simulink model "fullVehicleModel_17b"  (R2017b)
settings: Solver=VariableStepAuto  StartTime=0.0  StopTime=10.0  RelTol=1e-3
undefined symbols (not defined in the file): ambient_temp, bat, bat_r1, Batt, batt_initCharge, Batt_sensorLag_s, bvatt_AhRating, DiscIntNeverNeededParam, electronics_power, env, module_broad_area, module_small_area, module_top_area, mot, no_module, shifterPos, Ts, Ts_elec
libraries: Soft_ECUs x90, fl_lib x67, nesl_utility x29, Battery_lib x28, Gen_lib x13, simulink x10, aerolibconvert2 x7, SoftCAN_Interface x6, autolibshared x2, Additional_blocks_lib x1, elec_lib x1
(part 4 of 4)

== system fullVehicleModel_17b/Vehicle Model/Variant Subsystem/Subsystem/Battery Thermal/Module 5 ==
  Power Cycle : Inport
  Ideal Heat Flow Source : fl_lib/Thermal/Thermal Sources/Controlled Heat Flow Rate Source
      settings: SourceProductName=Simscape
  Ideal Temperature Sensor : fl_lib/Thermal/Thermal Sensors/Temperature Sensor
  Simulink-PS Converter1 : nesl_utility/Simulink-PS Converter  PhysicalDomain=network_engine_domain  SubClassName=ps_input  LeftPortType=input  RightPortType=output  PseudoPeriodic=off  Frequencies=[]  NoiseDistribution=none  NoiseParameters=[]  Unit=1  AffineConversion=off  FilteringAndDerivatives=zero  SimscapeFilterOrder=1  InputFilterTimeConstant=0.001  UdotUserProvided=1
  Thermal Mass : fl_lib/Thermal/Thermal Elements/Thermal Mass  mass=module_mass kg  sp_heat=specific_heat_module J/kg/K  T_specify=on  T_priority=High  T=ambient_temp K  T_nominal_specify=off  T_nominal_unit=K  T_nominal_value=1  Q_specify=off  Q_priority=High  Q=0 J/s  Q_nominal_specify=off  Q_nominal_unit=W  Q_nominal_value=1
  Thermal Reference1 : fl_lib/Thermal/Thermal Elements/Thermal Reference
  Thermal Reference2 : fl_lib/Thermal/Thermal Elements/Thermal Reference
  Temperature : PMIOPort  Port=1  Side=Right
  Air Convection : PMIOPort  Port=2  Side=Right
  Module to Module Convection : PMIOPort  Port=3  Side=Left
  Electronics to Module Convection : PMIOPort  Port=4  Side=Left
  wires:
  Power Cycle/1 -> Simulink-PS Converter1/1
  connections:
  Ideal Heat Flow Source/RConn1 -- Simulink-PS Converter1/RConn1
  Thermal Reference2/LConn1 -- Ideal Heat Flow Source/RConn2
  Temperature/RConn1 -- Ideal Temperature Sensor/RConn2
  Thermal Reference1/LConn1 -- Ideal Temperature Sensor/RConn1
  Ideal Heat Flow Source/LConn1 -- Module to Module Convection/RConn1 -- Electronics to Module Convection/RConn1 -- Ideal Temperature Sensor/LConn1 -- Thermal Mass/LConn1 -- Air Convection/RConn1

== system fullVehicleModel_17b/Vehicle Model/Variant Subsystem/Subsystem/Battery Thermal/Module 6 ==
  Power Cycle : Inport
  Ideal Heat Flow Source : fl_lib/Thermal/Thermal Sources/Controlled Heat Flow Rate Source
      settings: SourceProductName=Simscape
  Ideal Temperature Sensor : fl_lib/Thermal/Thermal Sensors/Temperature Sensor
  Simulink-PS Converter1 : nesl_utility/Simulink-PS Converter  PhysicalDomain=network_engine_domain  SubClassName=ps_input  LeftPortType=input  RightPortType=output  PseudoPeriodic=off  Frequencies=[]  NoiseDistribution=none  NoiseParameters=[]  Unit=1  AffineConversion=off  FilteringAndDerivatives=zero  SimscapeFilterOrder=1  InputFilterTimeConstant=0.001  UdotUserProvided=1
  Thermal Mass : fl_lib/Thermal/Thermal Elements/Thermal Mass  mass=module_mass kg  sp_heat=specific_heat_module J/kg/K  T_specify=on  T_priority=High  T=ambient_temp K  T_nominal_specify=off  T_nominal_unit=K  T_nominal_value=1  Q_specify=off  Q_priority=High  Q=0 J/s  Q_nominal_specify=off  Q_nominal_unit=W  Q_nominal_value=1
  Thermal Reference1 : fl_lib/Thermal/Thermal Elements/Thermal Reference
  Thermal Reference2 : fl_lib/Thermal/Thermal Elements/Thermal Reference
  Temperature : PMIOPort  Port=1  Side=Right
  Air Convection : PMIOPort  Port=2  Side=Right
  Convection from Module 7 : PMIOPort  Port=3  Side=Left
  Convection from Module 1 : PMIOPort  Port=4  Side=Left
  wires:
  Power Cycle/1 -> Simulink-PS Converter1/1
  connections:
  Ideal Heat Flow Source/RConn1 -- Simulink-PS Converter1/RConn1
  Thermal Reference2/LConn1 -- Ideal Heat Flow Source/RConn2
  Temperature/RConn1 -- Ideal Temperature Sensor/RConn2
  Thermal Reference1/LConn1 -- Ideal Temperature Sensor/RConn1
  Ideal Heat Flow Source/LConn1 -- Convection from Module 7/RConn1 -- Convection from Module 1/RConn1 -- Ideal Temperature Sensor/LConn1 -- Thermal Mass/LConn1 -- Air Convection/RConn1

== system fullVehicleModel_17b/Vehicle Model/Variant Subsystem/Subsystem/Battery Thermal/Module 7 ==
  Power Cycle : Inport
  Ideal Heat Flow Source : fl_lib/Thermal/Thermal Sources/Controlled Heat Flow Rate Source
      settings: SourceProductName=Simscape
  Ideal Temperature Sensor : fl_lib/Thermal/Thermal Sensors/Temperature Sensor
  Simulink-PS Converter1 : nesl_utility/Simulink-PS Converter  PhysicalDomain=network_engine_domain  SubClassName=ps_input  LeftPortType=input  RightPortType=output  PseudoPeriodic=off  Frequencies=[]  NoiseDistribution=none  NoiseParameters=[]  Unit=1  AffineConversion=off  FilteringAndDerivatives=zero  SimscapeFilterOrder=1  InputFilterTimeConstant=0.001  UdotUserProvided=1
  Thermal Mass : fl_lib/Thermal/Thermal Elements/Thermal Mass  mass=module_mass kg  sp_heat=specific_heat_module J/kg/K  T_specify=on  T_priority=High  T=ambient_temp K  T_nominal_specify=off  T_nominal_unit=K  T_nominal_value=1  Q_specify=off  Q_priority=High  Q=0 J/s  Q_nominal_specify=off  Q_nominal_unit=W  Q_nominal_value=1
  Thermal Reference1 : fl_lib/Thermal/Thermal Elements/Thermal Reference
  Thermal Reference2 : fl_lib/Thermal/Thermal Elements/Thermal Reference
  Temperature : PMIOPort  Port=1  Side=Right
  Air Convection : PMIOPort  Port=2  Side=Right
  Convection from Module 6 : PMIOPort  Port=3  Side=Left
  wires:
  Power Cycle/1 -> Simulink-PS Converter1/1
  connections:
  Ideal Heat Flow Source/RConn1 -- Simulink-PS Converter1/RConn1
  Thermal Reference2/LConn1 -- Ideal Heat Flow Source/RConn2
  Temperature/RConn1 -- Ideal Temperature Sensor/RConn2
  Thermal Reference1/LConn1 -- Ideal Temperature Sensor/RConn1
  Ideal Heat Flow Source/LConn1 -- Convection from Module 6/RConn1 -- Ideal Temperature Sensor/LConn1 -- Thermal Mass/LConn1 -- Air Convection/RConn1

== system fullVehicleModel_17b/Vehicle Model/Variant Subsystem/Subsystem/Output Signal Processing/Calculations ==
  note: unassigned vars
  A divide by hrs : fl_lib/Physical Signals/Functions/PS Gain  gain=-1/(60*60)
  Data Type Conversion : DataTypeConversion  OutDataTypeStr=fixdt(1,16,45)
  Data Type Conversion1 : DataTypeConversion  OutDataTypeStr=double
  Discrete-Time Integrator : DiscreteIntegrator  InitialCondition=batt_initCharge  SampleTime=Ts_elec  ICPrevOutput=DiscIntNeverNeededParam  ICPrevScaledInput=DiscIntNeverNeededParam
  PS Product : fl_lib/Physical Signals/Functions/PS Product
      settings: SourceProductName=Simscape
  PS-Simulink Converter{,1..3} (4 alike) : nesl_utility/PS-Simulink Converter  PhysicalDomain=network_engine_domain  SubClassName=ps_output  LeftPortType=input  RightPortType=output  PseudoPeriodic=off  Frequencies=[]  Unit=1  AffineConversion=off
  Terminator : Terminator
  W to KW : Gain  Gain=1/1000
  capacity to SOC : Gain  Gain=1/bvatt_AhRating * 100
  Voltage : PMIOPort  Port=1  Side=Left
  Current : PMIOPort  Port=2  Side=Left
  Batt_Ah : Outport
  Batt_SOC : Outport  Port=2
  Batt_Current : Outport  Port=3
  Batt_Voltage : Outport  Port=4
  wires:
  PS-Simulink Converter/1 -> W to KW/1
  W to KW/1 -> Terminator/1  "Batt_pwrElec_kW"
  PS-Simulink Converter1/1 -> Discrete-Time Integrator/1
  Discrete-Time Integrator/1 -> Data Type Conversion/1, Batt_Ah/1
  Data Type Conversion/1 -> Data Type Conversion1/1
  Data Type Conversion1/1 -> capacity to SOC/1
  capacity to SOC/1 -> Batt_SOC/1
  PS-Simulink Converter2/1 -> Batt_Current/1
  PS-Simulink Converter3/1 -> Batt_Voltage/1
  connections:
  Voltage/RConn1 -- PS-Simulink Converter3/LConn1 -- PS Product/LConn1
  Current/RConn1 -- PS-Simulink Converter2/LConn1 -- A divide by hrs/LConn1 -- PS Product/LConn2
  PS-Simulink Converter/LConn1 -- PS Product/RConn1
  PS-Simulink Converter1/LConn1 -- A divide by hrs/RConn1

== system fullVehicleModel_17b/Vehicle Model/Variant Subsystem/Subsystem/Output Signal Processing/SIgnal Processing ==
  note: 1) Add Subsystem or Model blocks as valid variant choices.
      | 2) You cannot connect blocks at this level. At simulation, connectivity is automatically
      | determined, based on the active variant and port name matching.
  Batt Temp : Inport
  Batt Capacity : Inport  Port=2
  Batt SOC : Inport  Port=3
  Batt Current : Inport  Port=4
  Batt Voltage : Inport  Port=5
  Subsystem : Subsystem  VariantControl=Variant
  Battery Measurements : Outport

== system fullVehicleModel_17b/Vehicle Model/Variant Subsystem1/Subsystem/Input Signal Processing/Subsystem ==
  note: Signal Selection
  HSC Inputs : Inport
  Genset : Inport  Port=2
  Driver : Inport  Port=3
  Signal Select : Subsystem
  Signal Select1 : Subsystem
  Singal Select2 : Subsystem
  DC Mode : Outport
  gen_loadTrq_Nm : Outport  Port=2
  gen_pwrElec_W : Outport  Port=3
  Aux Load : Outport  Port=4
  wires:
  Driver/1 -> Singal Select2/1(In1)
  Genset/1 -> Signal Select1/1(In1)
  HSC Inputs/1 -> Signal Select/1(In1)
  Singal Select2/1(Out1) -> Aux Load/1
  Signal Select1/2(Out2) -> gen_pwrElec_W/1
  Signal Select1/1(Out1) -> gen_loadTrq_Nm/1
  Signal Select/1(Out1) -> DC Mode/1

== system fullVehicleModel_17b/Controller Modules /Component Controllers/BMS Control Module/BMS Controller Module/EPO_Check/EPO_charge ==
  note: if the result is greater than the epo limit
      | then a fault is active
  note: and the resulting value is integrated until the current drops...
  note: then an output of -1 is multiplied with current^2...
  note: if the current is greater than max allowed...
  Current : Inport
  Chg_max_amps : Inport  Port=2
  Chg_max_plus_allowance : Inport  Port=3
  Chart : Stateflow chart  TreatAsAtomicUnit=on
  Constant : Constant  Value=bat.EPOintLimit
  Constant1 : Constant  Value=0
  Discrete-Time Integrator : DiscreteIntegrator  ExternalReset=level  InitialConditionSetting=State (most efficient)  SampleTime=Ts  ICPrevOutput=DiscIntNeverNeededParam  ICPrevScaledInput=DiscIntNeverNeededParam
  Math Function : Math  Operator=square  SaturateOnIntegerOverflow=on
  Product : Product
  Relational Operator : RelationalOperator  Operator===  OutDataTypeStr=boolean  RndMeth=Nearest
  Relational Operator1 : RelationalOperator  Operator=>  OutDataTypeStr=boolean  RndMeth=Nearest
  EPO : Outport
  wires:
  Constant1/1 -> Relational Operator/2
  Constant/1 -> Relational Operator1/2
  Relational Operator1/1 -> EPO/1
  Discrete-Time Integrator/1 -> Relational Operator1/1
  Product/1 -> Discrete-Time Integrator/1
  Chart/1(output) -> Product/1, Relational Operator/1
  Math Function/1 -> Product/2
  Chg_max_plus_allowance/1 -> Chart/2(max_plus_allowance)
  Relational Operator/1 -> Discrete-Time Integrator/2
  Chg_max_amps/1 -> Chart/3(max)
  Current/1 -> Chart/1(Current), Math Function/1

== system fullVehicleModel_17b/Controller Modules /Component Controllers/BMS Control Module/BMS Controller Module/EPO_Check/EPO_discharge ==
  note: see charge for comments
  Current : Inport
  max_discharge_plus_allowance : Inport  Port=2
  DIsChg_max_amps : Inport  Port=3
  Chart : Stateflow chart  TreatAsAtomicUnit=on
  Constant : Constant  Value=bat.EPOintLimit
  Constant1 : Constant  Value=0
  Discrete-Time Integrator : DiscreteIntegrator  ExternalReset=level  InitialConditionSetting=State (most efficient)  SampleTime=Ts  ICPrevOutput=DiscIntNeverNeededParam  ICPrevScaledInput=DiscIntNeverNeededParam
  Math Function : Math  Operator=square  SaturateOnIntegerOverflow=on
  Product : Product
  Relational Operator : RelationalOperator  Operator===  OutDataTypeStr=boolean  RndMeth=Nearest
  Relational Operator1 : RelationalOperator  Operator=>  OutDataTypeStr=boolean  RndMeth=Nearest
  EPO : Outport
  wires:
  Constant1/1 -> Relational Operator/2
  Relational Operator1/1 -> EPO/1
  Constant/1 -> Relational Operator1/2
  Discrete-Time Integrator/1 -> Relational Operator1/1
  Math Function/1 -> Product/2
  Relational Operator/1 -> Discrete-Time Integrator/2
  Product/1 -> Discrete-Time Integrator/1
  Chart/1(output) -> Product/1, Relational Operator/1
  DIsChg_max_amps/1 -> Chart/3(max)
  max_discharge_plus_allowance/1 -> Chart/2(max_plus_allowance)
  Current/1 -> Math Function/1, Chart/1(Current)

== system fullVehicleModel_17b/Controller Modules /Component Controllers/BMS Control Module/BMS Controller Module/Subsystem/Charge_Discharge_limit_maps ==
  bat_temp : Inport
  soc % : Inport  Port=2
  cclimit_map : Lookup_n-D  BreakpointsForDimension1=Batt.ChargeLimit.cont.temp  BreakpointsForDimension2=Batt.ChargeLimit.cont.soc  Table=Batt.ChargeLimit.cont.map  InternalRulePriority=Speed  RndMeth=Simplest  InputSameDT=on
  cplimit_map : Lookup_n-D  BreakpointsForDimension1=Batt.ChargeLimit.peak.temp  BreakpointsForDimension2=Batt.ChargeLimit.peak.soc  Table=Batt.ChargeLimit.peak.map  InternalRulePriority=Speed  RndMeth=Simplest  InputSameDT=on
  dclimit_map : Lookup_n-D  BreakpointsForDimension1=Batt.dichargeLimit.cont.temp  BreakpointsForDimension2=Batt.dichargeLimit.cont.soc  Table=Batt.dichargeLimit.cont.map  InternalRulePriority=Speed  RndMeth=Simplest  InputSameDT=on
  dplimit_map : Lookup_n-D  BreakpointsForDimension1=Batt.dichargeLimit.peak.temp  BreakpointsForDimension2=Batt.dichargeLimit.peak.soc  Table=Batt.dichargeLimit.peak.map  InternalRulePriority=Speed  RndMeth=Simplest  InputSameDT=on
  cplimit : Outport
  cclimit : Outport  Port=2
  dplimit : Outport  Port=3
  dclimit : Outport  Port=4
  wires:
  cclimit_map/1 -> cclimit/1
  dclimit_map/1 -> dclimit/1
  soc %/1 -> cplimit_map/2, cclimit_map/2, dplimit_map/2, dclimit_map/2
  bat_temp/1 -> cplimit_map/1, cclimit_map/1, dplimit_map/1, dclimit_map/1
  dplimit_map/1 -> dplimit/1
  cplimit_map/1 -> cplimit/1

== system fullVehicleModel_17b/Controller Modules /Component Controllers/Left Motor Control Module/Controller/Fault Daignosis/Device Temp to High ==
  Device Temp : Inport
  Compare To Constant : simulink/Logic and Bit Operations/Compare To Constant  relop=>  const=120  OutDataTypeStr=boolean
  Out1 : Outport
  wires:
  Compare To Constant/1 -> Out1/1
  Device Temp/1 -> Compare To Constant/1

== system fullVehicleModel_17b/Controller Modules /Component Controllers/Left Motor Control Module/Controller/Fault Daignosis/Motor Temp to High ==
  Mot_temp : Inport
  Compare To Constant : simulink/Logic and Bit Operations/Compare To Constant  relop=>  const=120  OutDataTypeStr=boolean
  Out1 : Outport
  wires:
  Mot_temp/1 -> Compare To Constant/1
  Compare To Constant/1 -> Out1/1

== system fullVehicleModel_17b/Controller Modules /Component Controllers/Left Motor Control Module/Controller/Fault Daignosis/No Power Supply Voltage ==
  mot_voltage : Inport
  Compare To Constant : simulink/Logic and Bit Operations/Compare To Constant  relop=<  const=24  OutDataTypeStr=boolean
  Out1 : Outport
  wires:
  Compare To Constant/1 -> Out1/1
  mot_voltage/1 -> Compare To Constant/1

== system fullVehicleModel_17b/Controller Modules /Component Controllers/Left Motor Control Module/Controller/Fault Daignosis/Over Current ==
  Motor Current : Inport
  Compare To Constant : simulink/Logic and Bit Operations/Compare To Constant  relop=>  const=800  OutDataTypeStr=boolean
  Out1 : Outport
  wires:
  Compare To Constant/1 -> Out1/1
  Motor Current/1 -> Compare To Constant/1

== system fullVehicleModel_17b/Controller Modules /Component Controllers/Left Motor Control Module/Controller/Fault Daignosis/Over Voltage ==
  Device Voltage : Inport
  Compare To Constant : simulink/Logic and Bit Operations/Compare To Constant  relop=>  const=1050  OutDataTypeStr=boolean
  Out1 : Outport
  wires:
  Compare To Constant/1 -> Out1/1
  Device Voltage/1 -> Compare To Constant/1

== system fullVehicleModel_17b/Vehicle Model/Variant Subsystem/Subsystem/Battery Thermal/Batt_overtemp_fault/First Degree Fault ==
  note: Mathematical Temp Model??
  Flag : Inport
  Temp : Inport  Port=2
  Power : Inport  Port=3
  Discrete-Time Integrator : DiscreteIntegrator  ExternalReset=level  InitialConditionSetting=State (most efficient)  SampleTime=Ts  ICPrevOutput=DiscIntNeverNeededParam  ICPrevScaledInput=DiscIntNeverNeededParam
  Gain : Gain  Gain=1/(30*30*bat_r1)
  Logical Operator : Logic  Operator=NOT  AllPortsSameDT=off  OutDataTypeStr=boolean
  Math Function : Math  SaturateOnIntegerOverflow=on
  Product : Product
  Product1 : Product
  Rate Transition : RateTransition
  Time_constant : Constant  Value=0.02
  Out1 : Outport
  wires:
  Logical Operator/1 -> Discrete-Time Integrator/2
  Discrete-Time Integrator/1 -> Product/1
  Rate Transition/1 -> Discrete-Time Integrator/1
  Power/1 -> Gain/1
  Product1/1 -> Out1/1
  Time_constant/1 -> Product/2
  Product/1 -> Math Function/1
  Math Function/1 -> Product1/2
  Gain/1 -> Rate Transition/1
  Flag/1 -> Logical Operator/1
  Temp/1 -> Product1/1

== system fullVehicleModel_17b/Vehicle Model/Variant Subsystem/Subsystem/Battery Thermal/Batt_overtemp_fault/Second Degree Fault ==
  In1 : Inport
  Constant : Constant  Value=0.005
  Memory : Memory
  Sum : Sum  Inputs=|++
  Out1 : Outport
  wires:
  Memory/1 -> Out1/1
  Sum/1 -> Memory/1
  Constant/1 -> Sum/2
  In1/1 -> Sum/1

== system fullVehicleModel_17b/Vehicle Model/Variant Subsystem/Subsystem/Output Signal Processing/SIgnal Processing/Subsystem ==
  note: Unit Conversion
  note: Scaling
  note: Sensor Lag
  Batt Capacity : Inport
  Batt SOC : Inport  Port=2
  Batt Current : Inport  Port=3
  Batt Voltage : Inport  Port=4
  Batt Temp : Inport  Port=5
  Bus Creator : BusCreator  Inputs=6
  Data Type Conversion{,1..5} (6 alike) : DataTypeConversion  OutDataTypeStr=double
  Gain : Gain  Gain=-1
  Power Post sensor : Product
  Sensor lag : Subsystem
  Sensor lag1 : Subsystem
  Battery Measurements : Outport
  wires:
  Batt Capacity/1 -> Data Type Conversion/1
  Data Type Conversion/1 -> Bus Creator/1  "Batt_battCapacity_Ah"
  Batt SOC/1 -> Data Type Conversion1/1
  Data Type Conversion1/1 -> Bus Creator/2  "Batt_SOC_pct"
  Sensor lag/1(Out1) -> Power Post sensor/1, Gain/1
  Sensor lag1/1(Out1) -> Power Post sensor/2, Data Type Conversion4/1
  Power Post sensor/1 -> Data Type Conversion3/1
  Batt Voltage/1 -> Sensor lag1/1(In1)
  Gain/1 -> Data Type Conversion2/1
  Batt Current/1 -> Sensor lag/1(In1)
  Batt Temp/1 -> Data Type Conversion5/1
  Data Type Conversion5/1 -> Bus Creator/6  "Batt_battTemp_C"
  Data Type Conversion4/1 -> Bus Creator/5  "Batt_voltage_V"
  Data Type Conversion3/1 -> Bus Creator/4  "Batt_battPwr_W"
  Data Type Conversion2/1 -> Bus Creator/3  "Batt_current_A"
  Bus Creator/1 -> Battery Measurements/1

== system fullVehicleModel_17b/Vehicle Model/Variant Subsystem1/Subsystem/Input Signal Processing/Subsystem/Signal Select ==
  In1 : Inport
  Bus Selector : BusSelector  OutputSignals=signal1
  Out1 : Outport
  wires:
  In1/1 -> Bus Selector/1
  Bus Selector/1 -> Out1/1  "<signal1>"

== system fullVehicleModel_17b/Vehicle Model/Variant Subsystem1/Subsystem/Input Signal Processing/Subsystem/Signal Select1 ==
  In1 : Inport
  Bus Selector : BusSelector  OutputSignals=signal1,signal2
  Out1 : Outport
  Out2 : Outport  Port=2
  wires:
  In1/1 -> Bus Selector/1
  Bus Selector/2 -> Out2/1  "<signal2>"
  Bus Selector/1 -> Out1/1  "<signal1>"

== system fullVehicleModel_17b/Vehicle Model/Variant Subsystem1/Subsystem/Input Signal Processing/Subsystem/Singal Select2 ==
  note: Auxiallary Power Load from driver
  In1 : Inport
  Bus Selector : BusSelector  OutputSignals=signal1
  Constant : Constant  Value=0
  From Workspace : FromWorkspace  VariableName=INV_accCurr_A  SampleTime=0
  Switch : Switch  Threshold=1
  Out1 : Outport
  wires:
  In1/1 -> Bus Selector/1
  Bus Selector/1 -> Switch/2  "<signal1>"
  Switch/1 -> Out1/1
  From Workspace/1 -> Switch/1
  Constant/1 -> Switch/3

== system fullVehicleModel_17b/Vehicle Model/Variant Subsystem/Subsystem/Output Signal Processing/SIgnal Processing/Subsystem/Sensor lag ==
  note: Create a sensor delay
      | efficient for small time delays
      | define delay in workspace (original value 0.01)
  In1 : Inport
  Discrete-Time Integrator : DiscreteIntegrator  InitialConditionSetting=State (most efficient)  SampleTime=1.000000000000000e-03  ICPrevOutput=DiscIntNeverNeededParam  ICPrevScaledInput=DiscIntNeverNeededParam
  Gain : Gain  Gain=1/Batt_sensorLag_s
  Sum : Sum  Inputs=|+-
  Out1 : Outport
  wires:
  In1/1 -> Sum/1
  Gain/1 -> Discrete-Time Integrator/1
  Discrete-Time Integrator/1 -> Out1/1, Sum/2
  Sum/1 -> Gain/1

== system fullVehicleModel_17b/Vehicle Model/Variant Subsystem/Subsystem/Output Signal Processing/SIgnal Processing/Subsystem/Sensor lag1 ==
  note: Create a sensor delay
      | efficient for small time delays
      | define delay in workspace (original value 0.01)
  In1 : Inport
  Discrete-Time Integrator : DiscreteIntegrator  InitialConditionSetting=State (most efficient)  SampleTime=1.000000000000000e-03  ICPrevOutput=DiscIntNeverNeededParam  ICPrevScaledInput=DiscIntNeverNeededParam
  Gain : Gain  Gain=1/Batt_sensorLag_s
  Sum : Sum  Inputs=|+-
  Out1 : Outport
  wires:
  In1/1 -> Sum/1
  Gain/1 -> Discrete-Time Integrator/1
  Discrete-Time Integrator/1 -> Out1/1, Sum/2
  Sum/1 -> Gain/1

== stateflow chart fullVehicleModel_17b/Controller Modules /Component Controllers/BMS Control Module/BMS Controller Module/EPO_Check/EPO_charge/Chart ==
  state less_than
    du: output = -1;
  state greater_than
    du: output = 1;
  state zero
    du: output = 0;
  less_than -> greater_than [order 1] : [Current > max_plus_allowance]
  greater_than -> less_than : [max_plus_allowance >= Current]
  less_than -> zero [order 2] : [Current < max]
  zero -> greater_than : [Current > max_plus_allowance]
  (default) -> zero
  data: Current input; max_plus_allowance input; output output; max input

== stateflow chart fullVehicleModel_17b/Controller Modules /Component Controllers/BMS Control Module/BMS Controller Module/EPO_Check/EPO_discharge/Chart ==
  state less_than
    du: output = -1;
  state greater_than
    du: output = 1;
  state zero
    du: output = 0;
  less_than -> greater_than [order 1] : [Current > max_plus_allowance]
  greater_than -> less_than : [max_plus_allowance >= Current]
  less_than -> zero [order 2] : [Current < max]
  zero -> greater_than : [Current > max_plus_allowance]
  (default) -> zero
  data: Current input; max_plus_allowance input; output output; max input

== stateflow chart fullVehicleModel_17b/Controller Modules /Component Controllers/BMS Control Module/BMS Controller Module/Startup Procedure ==
  state Startup
    du: bcm_veh_mon=1;
    ex: bcm_ready=1;
  state Wait_for_HSC_BCM_Enable
  state Wait
  state Inactive
    en: bcm_veh_mon=0;
    bcm_ready=0;
    bcm_cpwr_cmd=0;
    bcm_cpwr_mon=0;
  state Wait_for_Contactor_cmd
    du:
    bcm_cpwr_cmd=0;
    bcm_cpwr_mon=0;
  state Contactor_Power %Energize contactor actuator and wait
    du:
    bcm_cpwr_cmd = 1;
    bcm_cpwr_mon = 1;
  state Contactors_closed
  Wait_for_HSC_BCM_Enable -> Wait [order 2] : [hsc_bcm_enable==1]
  Startup -> Wait_for_HSC_BCM_Enable [order 2] : after (0.05, sec)[bcm_hvil_mon==1]
  (junction 46) -> Wait_for_HSC_BCM_Enable
  Wait -> (junction 46) [order 2] : [hsc_bcm_enable==0]
  Wait_for_Contactor_cmd -> (junction 46) [order 3] : [hsc_bcm_enable==0]
  Inactive -> Startup : [ignition>0]
  Startup -> Inactive [order 1] : [ignition==0]
  Wait_for_HSC_BCM_Enable -> (junction 44) [order 1] : [(bcm_hvil_mon==0)||(ignition==0)]
  Wait -> Wait_for_Contactor_cmd [order 1] : after (0.06, sec)
  (default) -> Inactive
  Contactors_closed -> Wait_for_Contactor_cmd : [(bcm_mainc_stat==0)||(bcm_hvil_mon==0)||(ignition==0)]
  (junction 44) -> Inactive
  Wait_for_Contactor_cmd -> (junction 44) [order 1] : [(bcm_hvil_mon==0)||(ignition==0)]
  Contactor_Power %Energize contactor actuator and wait -> Wait_for_Contactor_cmd [order 1] : [hsc_bcm_mainc_close==0]
  Wait_for_Contactor_cmd -> Contactor_Power %Energize contactor actuator and wait [order 2] : [hsc_bcm_mainc_close==1]
  Contactor_Power %Energize contactor actuator and wait -> Contactors_closed [order 2] : after(2,sec)[bcm_mainc_stat==1]
  data: hsc_bcm_mainc_close input; ignition input; bcm_hvil_mon input; bcm_veh_mon output; bcm_ready output; bcm_cpwr_mon output; bcm_cpwr_cmd output; hsc_bcm_enable input; bcm_mainc_stat input

== stateflow chart fullVehicleModel_17b/Controller Modules /Component Controllers/BMS Control Module/BMS Controller Module/contactor logic/Contactor_actuation ==
  state Close_Precharge
    du:
    Negative_actu = 0;
    Pre_charge_actu = 1;
    Positive_actu = 0;
  state Contactors_open
    du:
    Negative_actu = 0;
    Positive_actu = 0;
    Pre_charge_actu = 0;
  state Close_Negative
    du:
    Negative_actu = 1;
    Pre_charge_actu = 1;
    Positive_actu = 0;
  state Contactors_Closed
    du:
    Negative_actu = 1;
    Pre_charge_actu = 0;
    Positive_actu = 1;
  state Close_Positive
    du:
    Negative_actu = 1;
    Pre_charge_actu = 1;
    Positive_actu = 1;
  Contactors_open -> Close_Precharge : [close_contact == 1]
  Close_Precharge -> (junction 21) [order 1] : [close_contact == 1]
  (junction 21) -> Close_Negative : after(0.5,sec)
  Close_Precharge -> (junction 25) [order 2] : [close_contact == 0]
  (default) -> Contactors_open
  (junction 25) -> Contactors_open
  Close_Negative -> (junction 25) [order 1] : [close_contact == 0]
  Close_Positive -> (junction 25) [order 1] : [close_contact == 0]
  Close_Negative -> (junction 23) [order 2] : [close_contact == 1]
  Contactors_Closed -> Contactors_open : [close_contact == 0]
  Close_Positive -> Contactors_Closed [order 2] : after(0.85,sec)
  (junction 23) -> Close_Positive : after(0.5,sec)
  data: Negative_actu output; Positive_actu output; Pre_charge_actu output; close_contact input

== stateflow chart fullVehicleModel_17b/Controller Modules /Component Controllers/BMS Control Module/BMS Controller Module/contactor logic/EPO_Check ==
  state close_contactors
    du:
    contactors = 1;
  state open_contactors
    du:
    contactors = 0;
  (default) -> close_contactors
  open_contactors -> close_contactors : [EPO == 0 && contactor_rqst == 1]
  close_contactors -> open_contactors : [EPO == 1 || contactor_rqst == 0]
  data: EPO input; contactor_rqst input; contactors output

== stateflow chart fullVehicleModel_17b/Controller Modules /Component Controllers/INVCON Controller Module/INVCON Controller Module/INVCON Startup ==
  state Default
    en: SG_INV_State = 0;
  state State
    en: SG_INV_State = 1;
  state Transition
  (default) -> Default
  State -> Default : [(HV_voltage_V < 120)||(T15 == 0)]
  Default -> State [order 1] : [T15 == 1 && HV_voltage_V > 120]
  Default -> Transition [order 2] : [T15 == 1 && HV_voltage_V < 20]
  Transition -> State [order 1] : [HV_voltage_V >=120]
  Transition -> Default [order 2] : [T15 == 0]
  data: HV_voltage_V input; DCDC_ModeReq input; DC_Mode output

== stateflow chart fullVehicleModel_17b/Controller Modules /Component Controllers/Left Motor Control Module/Controller/REGID_Cycling ==
  state Send_btb
    en:
    mot_REGID=226;
  state Send_run
    en:
    mot_REGID=232;
  state Send_fault
    en:
    mot_REGID=143;
  state Send_currentAct
    en:
    mot_REGID=32;
  state Send_speedAct
    en:
    mot_REGID=48;
  (default) -> Send_btb
  Send_btb -> Send_run : after(10,msec)
  Send_run -> Send_currentAct : after(10,msec)
  Send_fault -> Send_btb : after(10,msec)
  Send_currentAct -> Send_speedAct : after(10,msec)
  (junction 62) -> Send_fault
  Send_speedAct -> (junction 62) : after(10,msec)
  data: mot_REGID output

== stateflow chart fullVehicleModel_17b/Controller Modules /Component Controllers/Left Motor Control Module/Controller/Startup_Shutdown_Procedure ==
  state EcuReady
    en:
    mot_btb = 1;
    mot_run = 0;
    mot_state = 0;
  state Off
    en:
    mot_state = 0;
    mot_run = 0;
    mot_btb = 0;
  state DriveReady
    en:
    mot_run = 1;
    mot_state = 0;
    mot_btb = 1;
  state ControllerEnable
    en:
    mot_state = 1;
    mot_run = 1;
    mot_btb = 1;
  (default) -> Off
  EcuReady -> DriveReady [order 1] : [mot_voltage>120]
  Off -> EcuReady : [ignition>0]
  EcuReady -> Off [order 2] : [ignition==0]
  DriveReady -> EcuReady [order 2] : [mot_voltage<120]
  ControllerEnable -> EcuReady [order 3] : [mot_voltage<120]
  DriveReady -> (junction 24) [order 3] : [ignition==0]
  (junction 24) -> Off
  ControllerEnable -> DriveReady [order 1] : [mot_mode == 0]
  DriveReady -> ControllerEnable [order 1] : [mot_mode ==1]
  ControllerEnable -> (junction 24) [order 2] : [ignition==0]
  data: mot_run output; mot_btb output; mot_state output; mot_mode input; ignition input; mot_voltage input
